simulink model "helicopter_LQR_tracking"  (R2021b)
settings: Solver=ode45  StartTime=0.0  StopTime=T  RelTol=1e-3
InitFcn:
  | hwinit
values from neighbouring files (symbols this model uses):
  adingain = [1 1 1 1]    [matlab.mat]
  adinoffs = [0 0 0 0]    [matlab.mat]
  h = 0.01    [calibration.m]    (also in controller1.m; controller_LQR.m; controller_LQR_trajectory.m; controller_pole_EKF.m)
undefined symbols (not defined in the file or in its folder): HeliMexHandle
libraries: simulink x1, sharedTrackingLibrary x1, eeGeneralControl x1, dspstat3 x1
settings Model: Creator=fkzhang  LastModifiedBy=lcaric
settings SolverCC: AlgebraicLoopSolver=TrustRegion
settings DataIOCC: LimitDataPoints=on  SaveFormat=Array  ReturnWorkspaceOutputs=off
settings OptimizationCC: BlockReduction=off  BooleanDataType=off  LifeSpan=inf
settings DebuggingCC: SaveWithParameterizedLinksMsg=none  UnderspecifiedInitializationDetection=Classic  MergeDetectMultiDrivingBlocksExec=none  SignalResolutionControl=TryResolveAllWithWarning  AllowSymbolicDim=off  SFUnexpectedBacktrackingDiag=warning  SFNoUnconditionalDefaultTransitionDiag=warning  SFExecutionAtInitializationDiag=none  SFMachineParentedDataDiag=warning  ArithmeticOperatorsInVariantConditions=warning
settings HardwareCC: ProdBitPerPointer=32  ProdBitPerSizeT=32  ProdBitPerPtrDiffT=32  ProdLargestAtomicFloat=None  ProdIntDivRoundTo=Undefined  ProdEndianess=Unspecified  ProdWordSize=32  ProdHWDeviceType=32-bit Generic  TargetUnknown=on
settings ModelReferenceCC: PropagateSignalLabelsOutOfModel=off
settings SFSimCC: SimUseLocalCustomCode=off  CustomCodeUndefinedFunction=UseInterfaceOnly
settings RTWCC: RTWUseLocalCustomCode=off
settings CodeAppCC: StateflowObjectComments=on
settings GRTTargetCC: TargetLangStandard=C89/C90 (ANSI)
settings ConfigComp: CovMetricSettings=dw  CovSaveCumulativeToWorkspaceVar=on  CovSaveSingleToWorkspaceVar=on  CovExternalEMLEnable=off  CovSFcnEnable=off

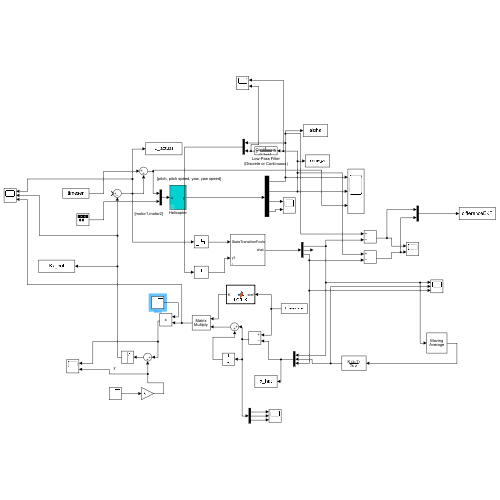
[thumbnail: Simulink's stored preview of the top-level diagram]
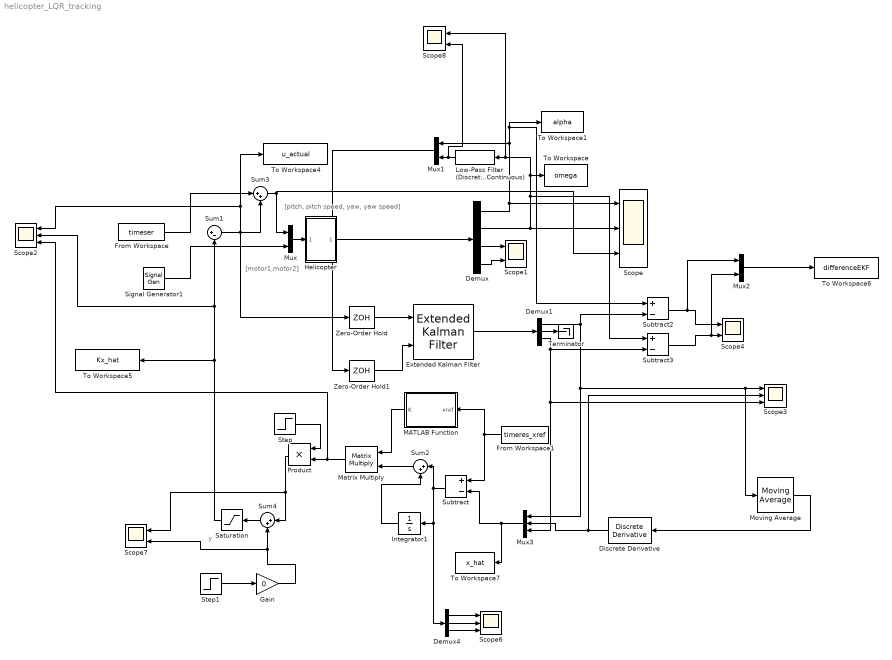
== system helicopter_LQR_tracking ==
  note: y
  note: [pitch, pitch speed, yaw, yaw speed]
  note: [motor1,motor2]
  Demux : Demux
  Demux1 : Demux  Outputs=3
  Demux4 : Demux  Outputs=3
  Discrete Derivative : simulink/Discrete/Discrete Derivative  gainval=1.0  ICPrevScaledInput=0.0  OutMin=[]  OutMax=[]  OutDataType=fixdt(1, 16)  OutScaling=2^-10  DoSatur=off
  Extended Kalman Filter : sharedTrackingLibrary/Extended Kalman Filter  StateTransitionFcn=nonlin_evolution  HasStateTransitionJacobianFcn=off  StateTransitionJacobianFcn=nonlin_jacobian  HasAdditiveProcessNoise=Additive  ProcessNoise=Q  HasTimeVaryingProcessNoise=off  HasStateTransitionFcnExtraArgument=1  InitialState=[0; 0; 0]  InitialStateCovariance=Q  MeasurementFcn1=nonlin_measurement_all  HasMeasurementJacobianFcn1=off  HasMeasurementEnablePort1=off  HasAdditiveMeasurementNoise1=Additive  MeasurementNoise1=R  HasTimeVaryingMeasurementNoise1=off  HasMeasurementFcnExtraArgument1=0  MeasurementFcn2=nonlin_measurement_omega  HasMeasurementJacobianFcn2=off  HasMeasurementEnablePort2=off  HasAdditiveMeasurementNoise2=Additive  MeasurementNoise2=10  HasTimeVaryingMeasurementNoise2=off  HasMeasurementFcnExtraArgument2=0  MeasurementFcn3=myMeasurementFcn  HasMeasurementJacobianFcn3=off  HasMeasurementEnablePort3=off  HasAdditiveMeasurementNoise3=Additive  MeasurementNoise3=1  HasTimeVaryingMeasurementNoise3=off  HasMeasurementFcnExtraArgument3=0  MeasurementFcn4=myMeasurementFcn  HasMeasurementJacobianFcn4=off  HasMeasurementEnablePort4=off  HasAdditiveMeasurementNoise4=Additive  MeasurementNoise4=1  HasTimeVaryingMeasurementNoise4=off  HasMeasurementFcnExtraArgument4=0  MeasurementFcn5=myMeasurementFcn  HasMeasurementJacobianFcn5=off  HasMeasurementEnablePort5=off  HasAdditiveMeasurementNoise5=Additive  MeasurementNoise5=1  HasTimeVaryingMeasurementNoise5=off  HasMeasurementFcnExtraArgument5=0  EnableMultirate=off  StateTransitionFcnSampleTime=1  MeasurementFcn1SampleTime=1  MeasurementFcn2SampleTime=1  MeasurementFcn3SampleTime=1  MeasurementFcn4SampleTime=1  MeasurementFcn5SampleTime=1  UseCurrentEstimator=on  OutputStateCovariance=off  DataType=double  SampleTime=0.02  NumberOfMeasurements=1
      settings: SourceProductBaseCode=AE,PW,CT,DR,TF,ID,LP,NV,AR,RO,RR,UV,VE
  From Workspace : FromWorkspace  VariableName=timeser
  From Workspace1 : FromWorkspace  VariableName=timeres_xref
  Gain : Gain  Gain=0
  Helicopter : Subsystem  mask{Ts=h}
      mask prompts: Ts "sampletime"
      mask init:
      | sf_heli_init
      mask Display:
      | port_label('input',1,'u');
      | port_label('output',1,'y');
  Integrator1 : Integrator
  Low-Pass Filter (Discrete or Continuous) : eeGeneralControl/Low-Pass Filter (Discrete or Continuous)  K=1  T=0.1  B=inf  A=-inf  init_option=Inherited from block input  x0=0  Ts=0
  MATLAB Function : MATLAB Function  TreatAsAtomicUnit=on
  Matrix Multiply : Product  Multiplication=Matrix(*)
  Moving Average : dspstat3/Moving Average  Method=Sliding window  ForgettingFactorPort=off  SpecifyWindowLength=on  WindowLength=5  ForgettingFactor=0.9  SimulateUsing=Code generation
  Mux : Mux  Inputs=2
  Mux1 : Mux  Inputs=2
  Mux2 : Mux  Inputs=2
  Mux3 : Mux  Inputs=3
  Product : Product
  Saturation : Saturate  UpperLimit=1  LowerLimit=-1
  Scope{,2..3,6} (4 alike) : Scope  NumInputPorts=3
  Scope{1,4,7..8} (4 alike) : Scope  NumInputPorts=2
  Signal Generator1 : SignalGenerator  WaveForm=square  Amplitude=0  Frequency=1/20
  Step : Step  Time=0  Before=1  SampleTime=0
  Step1 : Step  After=0  SampleTime=0
  Subtract : Sum  Inputs=+-
  Subtract2 : Sum  Inputs=+-
  Subtract3 : Sum  Inputs=+-
  Sum1 : Sum  Inputs=|+-
  Sum2 : Sum  Inputs=|++
  Sum3 : Sum  Inputs=|++
  Sum4 : Sum  Inputs=|++
  Terminator : Terminator
  To Workspace : ToWorkspace  VariableName=omega  SaveFormat=Timeseries  SampleTime=-1
  To Workspace1 : ToWorkspace  VariableName=alpha  SaveFormat=Timeseries  SampleTime=-1
  To Workspace4 : ToWorkspace  VariableName=u_actual  SaveFormat=Timeseries  SampleTime=-1
  To Workspace5 : ToWorkspace  VariableName=Kx_hat  SaveFormat=Timeseries  SampleTime=-1
  To Workspace6 : ToWorkspace  VariableName=differenceEKF  SaveFormat=Timeseries  SampleTime=-1
  To Workspace7 : ToWorkspace  VariableName=x_hat  SaveFormat=Timeseries  SampleTime=-1
  Zero-Order Hold : ZeroOrderHold  SampleTime=0.02
  Zero-Order Hold1 : ZeroOrderHold  SampleTime=0.02
  wires:
  Mux/1 -> Helicopter/1(In1)
  Signal Generator1/1 -> Mux/2
  Demux/2 -> Scope8/1, Low-Pass Filter (Discrete or Continuous)/1, To Workspace/1, Subtract3/1, Scope/2
  Demux/3 -> Scope1/1
  Demux/4 -> Scope1/2
  From Workspace/1 -> Sum3/1
  Demux/1 -> Subtract2/1, To Workspace1/1, Mux1/1, Scope/1
  Mux1/1 -> Zero-Order Hold1/1
  Helicopter/1(Out1) -> Demux/1
  Sum1/1 -> Sum3/2, To Workspace4/1, Scope2/1, Zero-Order Hold/1
  MATLAB Function/1(K) -> Matrix Multiply/1
  Saturation/1 -> To Workspace5/1, Scope2/2, Sum1/2
  From Workspace1/1 -> Subtract/1, MATLAB Function/1(xref)
  Sum2/1 -> Matrix Multiply/2
  Zero-Order Hold/1 -> Extended Kalman Filter/1
  Zero-Order Hold1/1 -> Extended Kalman Filter/2
  Extended Kalman Filter/1 -> Demux1/1
  Demux1/3 -> Subtract3/2, Mux3/3, Scope3/3
  Subtract2/1 -> Scope4/1, Mux2/1
  Subtract3/1 -> Mux2/2, Scope4/2
  Mux2/1 -> To Workspace6/1
  Low-Pass Filter (Discrete or Continuous)/1 -> Scope8/2, Mux1/2
  Demux1/1 -> Subtract2/2, Mux3/1, Moving Average/1, Scope3/1
  Discrete Derivative/1 -> Scope3/2, Mux3/2
  Mux3/1 -> To Workspace7/1, Subtract/2
  Moving Average/1 -> Discrete Derivative/1
  Step/1 -> Product/1
  Product/1 -> Scope7/1, Sum4/1
  Sum4/1 -> Saturation/1
  Step1/1 -> Gain/1
  Gain/1 -> Scope7/2, Sum4/2
  Demux1/2 -> Terminator/1
  Demux4/1 -> Scope6/1
  Demux4/3 -> Scope6/3
  Demux4/2 -> Scope6/2
  Subtract/1 -> Integrator1/1, Demux4/1, Sum2/1
  Integrator1/1 -> Sum2/2
  Matrix Multiply/1 -> Scope2/3, Product/2
  Sum3/1 -> Mux/1, Scope/3

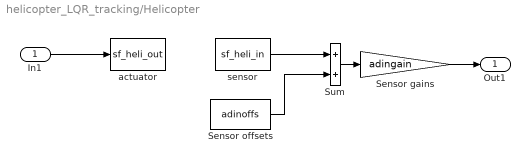
== system helicopter_LQR_tracking/Helicopter ==
  In1 : Inport
  Sensor gains : Gain  Gain=adingain
  Sensor offsets : Constant  Value=adinoffs
  Sum : Sum
  actuator : M-S-Function  FunctionName=sf_heli_out  Parameters=HeliMexHandle,Ts
  sensor : M-S-Function  FunctionName=sf_heli_in  Parameters=HeliMexHandle
  Out1 : Outport  VectorParamsAs1DForOutWhenUnconnected=off
  wires:
  sensor/1 -> Sum/1
  In1/1 -> actuator/1
  Sensor offsets/1 -> Sum/2
  Sum/1 -> Sensor gains/1
  Sensor gains/1 -> Out1/1

== matlab function helicopter_LQR_tracking/MATLAB Function ==
  data: xref input; K output
function K = LQR_K(xref)
coder.extrinsic('get_K_tracking');
K1 = 0;
K3 = 0;
K4 = 0;
b = 0;
C = [1, 0, 0; 0, 0, 1];

% choose alpha -> calc omega
if xref(1) <= 0
    b = 0.239927543450809;
    K1 = -10.548800723683954;
    K3 = 5.498506290874219e-05;
    K4 = 4.594429729616914;
%   f_u = 272.9 * u * u + 593.4 * u - 8.529;
else
    b = 0.025936940902745;
    K1 = -10.577796958770156;
    K3 = -2.433475804656021e-05;
    K4 = 5.379206715771331;
%     f_u = -284.3 * u * u + 609 * u + 7.086;
end

Q_lqr=zeros(3);
R_lqr=[0];
N=0;

alpha_ref = xref(1);
if alpha_ref>0 && alpha_ref<0.1
Q_lqr = [3500, 0, 0; 0, 20, 0; 0, 0, 0.03];
R_lqr = [5];
N = 0;
%x_ref = [alpha_ref; alpha_dot_ref; omega_ref]/1;
elseif alpha_ref>=0.1 && alpha_ref<0.2
Q_lqr = [1000, 0, 0; 0, 20, 0; 0, 0, 0.03];
R_lqr = [5];
N = 0;
%x_ref = [alpha_ref; alpha_dot_ref; omega_ref]/0.9;
elseif alpha_ref>=0.2
Q_lqr = [2000, 0, 0; 0, 20, 0; 0, 0, 0.05];
R_lqr = [5];
N = 0;
%x_ref = [alpha_ref; alpha_dot_ref; omega_ref]/0.99;
elseif alpha_ref<0 && alpha_ref>-0.2
Q_lqr = [5000, 0, 0; 0, 20, 0; 0, 0, 0.1];
R_lqr = [8];
N = 0;
elseif alpha_ref>=-0.4
Q_lqr = [2000, 0, 0; 0, 5, 0; 0, 0, 0.1];
R_lqr = [8];
N = 0;
%x_ref = [alpha_ref; alpha_dot_ref; omega_ref]/0.9;
elseif alpha_ref<-0.4
Q_lqr = [2000, 0, 0; 0, 30, 0; 0, 0, 0.1];
R_lqr = [8];
N = 0;
%x_ref = [alpha_ref; alpha_dot_ref; omega_ref]/0.9;
end
[A_lin,B_lin] = observer_simulink(xref(1));
K=zeros(1,3);
K = get_K_tracking(A_lin, B_lin,Q_lqr,R_lqr);
